simulink model "untitled"  (R2025a)
settings: Solver=VariableStepAuto  StartTime=0.0  StopTime=100  RelTol=1e-3
libraries: SignalEditorBlockLib x1
settings Model: Creator=mefat  LastModifiedBy=mefat

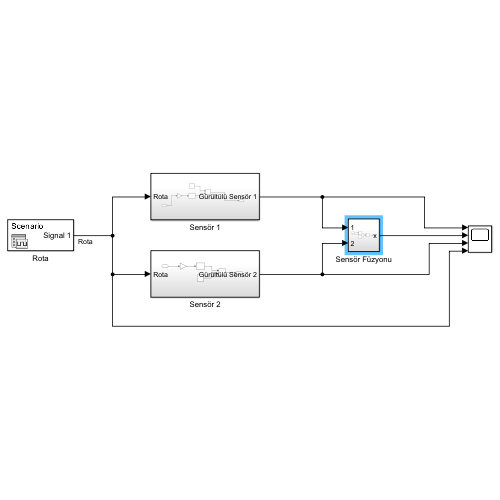
[thumbnail: Simulink's stored preview of the top-level diagram]
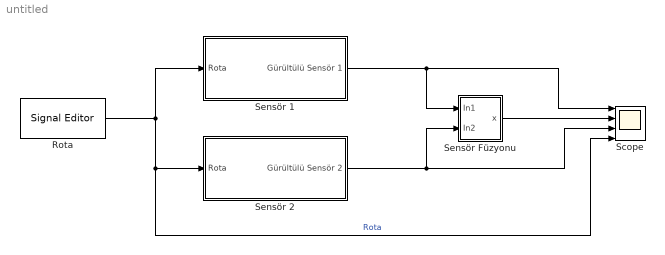
== system untitled ==
  Rota : SignalEditorBlockLib/Signal Editor  FileName=untitled.mat  ActiveScenario=Scenario  ActiveSignal=Signal 1  IsBus=off  OutputBusObjectStr=Bus: BusObject  SampleTime=0.01  ZeroCross=off  OutputAfterFinalValue=Setting to zero  Unit=m  PreserveSignalName=on  ApplySigPropsToAllScenarios=off  ApplySigPropsToAllSignals=off  SignalPropertySource=Dialog parameters
  Scope : Scope  NumInputPorts=4
      settings: ActiveDisplayYMinimum=-5.2071706376905018  ActiveDisplayYMaximum=27.092254677562277
  Sensör 1 : Subsystem
  Sensör 2 : Subsystem
  Sensör Füzyonu : Subsystem
  wires:
  Sensör 1/1(Gürültülü Sensör 1) -> Sensör Füzyonu/1(In1), Scope/1
  Sensör 2/1(Gürültülü Sensör 2) -> Sensör Füzyonu/2(In2), Scope/3
  Sensör Füzyonu/1(x) -> Scope/2
  Rota/1 -> Scope/4, Sensör 2/1(Rota), Sensör 1/1(Rota)  "Rota"

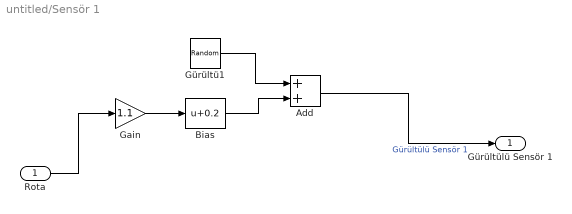
== system untitled/Sensör 1 ==
  Rota : Inport
  Add : Sum
  Bias : Bias  Bias=0.2  SaturateOnIntegerOverflow=off
  Gain : Gain  Gain=1.1
  Gürültü1 : RandomNumber  SampleTime=0.1
  Gürültülü Sensör 1 : Outport
  wires:
  Gürültü1/1 -> Add/1
  Gain/1 -> Bias/1
  Bias/1 -> Add/2
  Rota/1 -> Gain/1
  Add/1 -> Gürültülü Sensör 1/1  "Gürültülü Sensör 1"

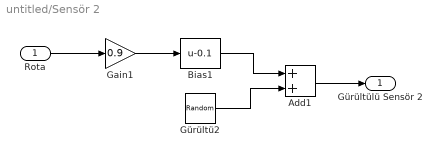
== system untitled/Sensör 2 ==
  Rota : Inport
  Add1 : Sum
  Bias1 : Bias  Bias=-0.1  SaturateOnIntegerOverflow=off
  Gain1 : Gain  Gain=0.9
  Gürültü2 : RandomNumber  Variance=2  SampleTime=0.1
  Gürültülü Sensör 2 : Outport
  wires:
  Gain1/1 -> Bias1/1
  Gürültü2/1 -> Add1/2
  Bias1/1 -> Add1/1
  Rota/1 -> Gain1/1
  Add1/1 -> Gürültülü Sensör 2/1

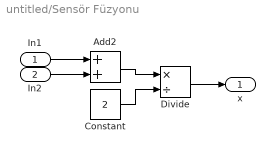
== system untitled/Sensör Füzyonu ==
  In1 : Inport
  In2 : Inport  Port=2
  Add2 : Sum
  Constant : Constant  Value=2
  Divide : Product  Inputs=*/
  x : Outport
  wires:
  Constant/1 -> Divide/2
  Add2/1 -> Divide/1
  In2/1 -> Add2/2
  Divide/1 -> x/1
  In1/1 -> Add2/1
